simulink model "AS1_Un_Balanced_load_7bus"  (R2021a)
settings: Solver=ode45  StartTime=0.0  StopTime=1  RelTol=1e-3  EnableMultiTasking=on
undefined symbols (not defined in the file): D11, Delta
libraries: spsDCVoltageSourceLib x12, spsDiodeLib x12, spsSeriesRLCBranchLib x12, spsGroundLib x9, spsThreePhaseTransformerTwoWindingsLib x7, spsBreakerLib x7, spsThreePhaseParallelRLCLoadLib x6, simulink_extras x6, spsThreePhaseSeriesRLCBranchLib x6, dspstat3 x3, spsThreePhaseVIMeasurementLib x3, spsCurrentMeasurementLib x2
settings Model: Creator=Gajanan-pc  LastModifiedBy=sony
settings SolverCC: AlgebraicLoopSolver=TrustRegion
settings DataIOCC: LimitDataPoints=on  SaveFormat=Array  ReturnWorkspaceOutputs=off
settings OptimizationCC: LifeSpan=inf
settings DebuggingCC: MaxConsecutiveZCsMsg=none  SolverPrmCheckMsg=warning  ParameterPrecisionLossMsg=none  SFUnexpectedBacktrackingDiag=warning  SFNoUnconditionalDefaultTransitionDiag=warning  SFExecutionAtInitializationDiag=none  SFMachineParentedDataDiag=warning  ArithmeticOperatorsInVariantConditions=warning
settings HardwareCC: ProdBitPerPointer=32  ProdBitPerSizeT=32  ProdBitPerPtrDiffT=32  ProdLargestAtomicFloat=None  ProdIntDivRoundTo=Undefined  ProdEndianess=Unspecified  ProdWordSize=32  ProdHWDeviceType=32-bit Generic
settings ModelReferenceCC: PropagateSignalLabelsOutOfModel=off
settings SFSimCC: SimUseLocalCustomCode=off  CustomCodeUndefinedFunction=UseInterfaceOnly
settings RTWCC: RTWUseLocalCustomCode=off
settings CodeAppCC: StateflowObjectComments=on
settings GRTTargetCC: TargetLangStandard=C89/C90 (ANSI)
settings ConfigComp: CovMetricSettings=dw  CovSaveCumulativeToWorkspaceVar=on  CovSaveSingleToWorkspaceVar=on  CovExternalEMLEnable=off  CovSFcnEnable=off
settings SimscapeCC: SimscapeNormalizeSystem=off

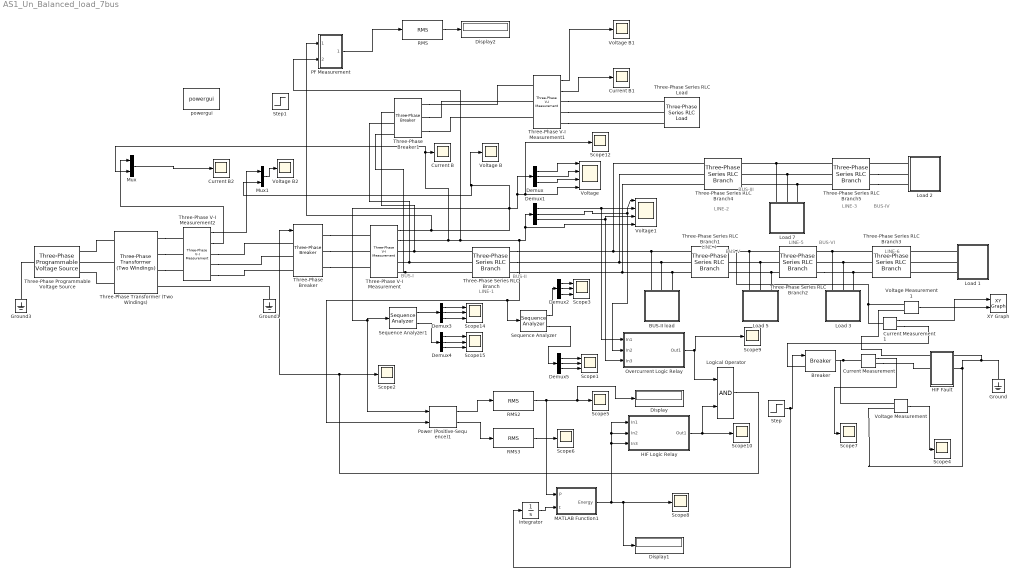
== system AS1_Un_Balanced_load_7bus ==
  note: LINE-1
  note: BUS-I
  note: BUS-II
  note: BUS-III
  note: BUS-IV
  note: BUS-V
  note: BUS-VI
  note: LINE-2
  note: LINE-3
  note: LINE-4
  note: LINE-5
  note: LINE-6
  BUS-II load : Subsystem
  Breaker : spsBreakerLib/Breaker  InitialState=0  SwitchingTimes="[1/50  5/50]"  External=on  BreakerResistance=0.01  SnubberResistance=1e6  SnubberCapacitance=inf  Measurements=Branch voltage and current  MoreParameters=on  NoBreakLoop=off
      settings: SourceProductBaseCode=PS
  Current B : Scope
  Current B1 : Scope
  Current B2 : Scope
  Current Measurement : spsCurrentMeasurementLib/Current Measurement  PhasorSimulation=off  OutputType=Complex  PSBequivalent=0
  Current Measurement1 : spsCurrentMeasurementLib/Current Measurement  PhasorSimulation=off  OutputType=Complex  PSBequivalent=0
  Demux{,1..5} (6 alike) : Demux  Outputs=3
  Display : Display
  Display1 : Display
  Display2 : Display
  Ground : spsGroundLib/Ground  LConnTagsString=a
  Ground1 : spsGroundLib/Ground  LConnTagsString=a
  Ground3 : spsGroundLib/Ground  LConnTagsString=a
  HIF Fault : Subsystem
  HIF Logic Relay : Subsystem  TreatAsAtomicUnit=on
  Integrator : Integrator
  Load 1 : Subsystem
  Load 2 : Subsystem
  Load 3 : Subsystem
  Load 5 : Subsystem
  Load 7 : Subsystem
  Logical Operator : Logic  AllPortsSameDT=off
  MATLAB Function1 : MATLAB Function  TreatAsAtomicUnit=on
  Mux : Mux  Inputs=2
  Mux1 : Mux  Inputs=2
  Overcurrent Logic Relay : Subsystem  TreatAsAtomicUnit=on
  PF Measurement : Subsystem
  Power (Positive-Sequence)1 : spsPowerPositiveSequenceLib/Power (Positive-Sequence)  Freq=50  Vinit=[0, 0]  Iinit=[0, 0]  Ts=0
      link override Sequence Analyzer: Freq=50  seq=Negative
      link override Sequence Analyzer1: Freq=50  seq=Zero
      settings: SourceProductBaseCode=PS
  RMS : dspstat3/RMS  run=off  directionMode=Each column  dimension=1  InputProcessing=Columns as channels (frame based)  reset_popup=None
  RMS2 : dspstat3/RMS  run=off  directionMode=Each column  dimension=1  InputProcessing=Columns as channels (frame based)  reset_popup=None
  RMS3 : dspstat3/RMS  run=off  directionMode=Each column  dimension=1  InputProcessing=Columns as channels (frame based)  reset_popup=None
  Scope{1,3,14..15} (4 alike) : Scope  NumInputPorts=3
  Scope{2,4..10,12} (9 alike) : Scope
  Sequence Analyzer : spsSequenceAnalyzerLib/Sequence Analyzer  Freq=50  n=1  seq=Positive Negative Zero  InInit=[1, 0]  Ts=0
      link override Fourier_A: Freq=50
      link override Fourier_B: Freq=50
      link override Fourier_C: Freq=50
      settings: SourceProductBaseCode=PS
  Sequence Analyzer1 : spsSequenceAnalyzerLib/Sequence Analyzer  Freq=50  n=1  seq=Positive Negative Zero  InInit=[1, 0]  Ts=0
      link override Fourier_A: Freq=50
      link override Fourier_B: Freq=50
      link override Fourier_C: Freq=50
      settings: SourceProductBaseCode=PS
  Step : Step  Time=0.9  SampleTime=0.1  ZeroCross=off
  Step1 : Step  Time=0.8  SampleTime=0.1  ZeroCross=off
  Three-Phase Programmable Voltage Source : spsThreePhaseProgrammableVoltageSourceLib/Three-Phase Programmable Voltage Source  PositiveSequence="[33e3  0 50]"  VariationEntity=None  VariationType=Table of time-amplitude pairs  VariationTypeAlt=Step  VariationStep=0.5  VariationRate=10  VariationMagnitude=0.3  VariationFrequency=2  VariationTiming=[.01 .05 1]  VariationPhaseA=off  Amplitudes=[1 0.8 1.2 1.0]  TimeValues=[0 0.1 0.15 0.2]  HarmonicGeneration=off  HarmonicA=[3 0.2 -25 0]  HarmonicB=[2 0.15 35 2]  Timing="[0.05  3]"  BusType=PQ  Pref=5e6  Qref=0  Qmin=0.5e6  Qmax=0
  Three-Phase Series RLC Branch : spsThreePhaseSeriesRLCBranchLib/Three-Phase Series RLC Branch  LConnTagsString=A|B|C  RConnTagsString=A|B|C  BranchType=RL  Resistance=0.2232  Inductance=0.012  Capacitance=0  Measurements=None
  Three-Phase Series RLC Branch1 : spsThreePhaseSeriesRLCBranchLib/Three-Phase Series RLC Branch  LConnTagsString=A|B|C  RConnTagsString=A|B|C  BranchType=RL  Resistance=0.9207  Inductance=0.0495  Capacitance=0  Measurements=None
  Three-Phase Series RLC Branch2 : spsThreePhaseSeriesRLCBranchLib/Three-Phase Series RLC Branch  LConnTagsString=A|B|C  RConnTagsString=A|B|C  BranchType=RL  Resistance=0.6138  Inductance=0.33  Capacitance=0  Measurements=None
  Three-Phase Series RLC Branch3 : spsThreePhaseSeriesRLCBranchLib/Three-Phase Series RLC Branch  LConnTagsString=A|B|C  RConnTagsString=A|B|C  BranchType=RL  Resistance=1.602  Inductance=0.057  Capacitance=0  Measurements=None
  Three-Phase Series RLC Branch4 : spsThreePhaseSeriesRLCBranchLib/Three-Phase Series RLC Branch  LConnTagsString=A|B|C  RConnTagsString=A|B|C  BranchType=RL  Resistance=0.7812  Inductance=0.042  Capacitance=0  Measurements=None
  Three-Phase Series RLC Branch5 : spsThreePhaseSeriesRLCBranchLib/Three-Phase Series RLC Branch  LConnTagsString=A|B|C  RConnTagsString=A|B|C  BranchType=RL  Resistance=1.1997  Inductance=0.0645  Capacitance=0  Measurements=None
  Three-Phase Series RLC Load : spsThreePhaseSeriesRLCLoadLib/Three-Phase Series RLC Load  LConnTagsString=A|B|C  Configuration=Y (floating)  NominalVoltage=12e3  Vabc=[1e3 1e3 1e3]  Vabcp=[1e3 1e3 1e3]  NominalFrequency=50  UnbalancedPower=off  ActivePower=0  InductivePower=18e3  CapacitivePower=1800e3  Pabc=[10e3 9e3 11e3]  QLabc=[100 90 110]  QCabc=[100 90 110]  Pabcp=[10e3 9e3 11e3]  QLabcp=[100 90 110]  QCabcp=[100 90 110]  Measurements=Branch voltages and currents  LoadType=constant Z
  Three-Phase Transformer (Two Windings) : spsThreePhaseTransformerTwoWindingsLib/Three-Phase Transformer (Two Windings)  Winding1Connection=Delta (D11)  Winding2Connection=Yn  CoreType=Three-limb core (core-type)  SetSaturation=off  Hysteresis=off  DataFile='hysteresis'  SetInitialFlux=off  Measurements=None  UNITS=pu  NominalPower=[ 10e6 , 50 ]  Winding1=[33e3 , 0.002 , 0.08 ]  Winding2=[11e3 , 0.002 , 0.08 ]  Rm=500  Lm=500  L0=0.5  Saturation=[ 0,0 ; 0.0024,1.2 ; 1.0,1.52 ]  InitialFluxes=[-0.84855560977397 0.870082768362299 -0.0215271585931069]  BreakLoop=off  DiscreteSolver=Trapezoidal iterative  DataType=off  TransfoNumber=1
  Three-Phase V-I Measurement : spsThreePhaseVIMeasurementLib/Three-Phase V-I Measurement  VoltageMeasurement=phase-to-phase  SetLabelV=off  LabelV=Vabc  Vpu=off  VpuLL=off  CurrentMeasurement=yes  SetLabelI=off  LabelI=Iabc  Ipu=off  Pbase=100e6  Vbase=11e3  OutputType=Complex  PhasorSimulation=off  PSBequivalent=0
  Three-Phase V-I Measurement1 : spsThreePhaseVIMeasurementLib/Three-Phase V-I Measurement  VoltageMeasurement=phase-to-phase  SetLabelV=off  LabelV=Vabc  Vpu=off  VpuLL=off  CurrentMeasurement=yes  SetLabelI=off  LabelI=Iabc  Ipu=off  Pbase=100e6  Vbase=11e3  OutputType=Complex  PhasorSimulation=off  PSBequivalent=0
  Three-Phase V-I Measurement2 : spsThreePhaseVIMeasurementLib/Three-Phase V-I Measurement  VoltageMeasurement=phase-to-phase  SetLabelV=off  LabelV=Vabc  Vpu=off  VpuLL=off  CurrentMeasurement=yes  SetLabelI=off  LabelI=Iabc  Ipu=off  Pbase=100e6  Vbase=11e3  OutputType=Complex  PhasorSimulation=off  PSBequivalent=0
  Three-Phase Breaker : spsThreePhaseBreakerLib/Three-Phase Breaker  InitialState=closed  SwitchA=on  SwitchB=on  SwitchC=on  SwitchTimes=[1/50 5/50]  External=on  BreakerResistance=0.01  SnubberResistance=1e6  SnubberCapacitance=inf  Measurements=Breaker voltages and currents
  Three-Phase Breaker1 : spsThreePhaseBreakerLib/Three-Phase Breaker  InitialState=closed  SwitchA=on  SwitchB=on  SwitchC=on  SwitchTimes=[1/50 5/50]  External=on  BreakerResistance=0.01  SnubberResistance=1e6  SnubberCapacitance=inf  Measurements=Breaker voltages and currents
  Voltage : Scope  NumInputPorts=4
  Voltage B : Scope
  Voltage B1 : Scope
  Voltage B2 : Scope
  Voltage Measurement : spsVoltageMeasurementLib/Voltage Measurement  PhasorSimulation=off  OutputType=Complex  PSBequivalent=0
  Voltage Measurement1 : spsVoltageMeasurementLib/Voltage Measurement  PhasorSimulation=off  OutputType=Complex  PSBequivalent=0
  Voltage1 : Scope  NumInputPorts=4
  XY Graph : simulink/Sinks/XY Graph  xmin=-100  xmax=100  ymin=-7000  ymax=7000  st=-1
  powergui : spspowerguiLib/powergui  Priority=1  SimulationMode=Discrete  SampleTime=50e-6  frequency=60  Iterations=50  frequencyindice=0  Pbase=100e6  ErrMax=0.0001  UnitsV=kV  UnitsW=MW  buscounter=0  FunctionMessages=off  echomessages=off  EnableUseOfTLC=off  CurrentSourceSwitches=off  DisableSnubberDevices=off  DisableRonSwitches=off  DisableVfSwitches=off  DisplayEquations=off  AutomaticDiscreteSolvers=off  SolverType=Backward Euler  Interpol=off  ExternalGateDelay=off  methode=off  Ts=0  x0status=blocks  SPID=off  SwTol=0  HookPort=off  NonlinearTolerance=0  nMaxIteration=15  ContinueOnMaxIteration=off  RestoreLinks=warning  ResistiveCurrentMeasurement=off  Frange=[0:2:500]  Ylog=off  Xlog=on  ShowGrid=off  save=off  variable=ZData  structure=0  ZoomFFT=off  StartTime=0.0  cycles=1  DisplayStyle=1  fundamental=60  FreqAxis=off  MaxFrequency=1000  frequencyindicesteady=1  RmsSteady=1  display=off
  wires:
  Demux1/3 -> Voltage1/3, Overcurrent Logic Relay/3(In3)
  Demux/1 -> Voltage/1
  Demux/2 -> Voltage/2
  Demux/3 -> Voltage/3
  Demux1/2 -> Voltage1/2, Overcurrent Logic Relay/2(In2)
  Three-Phase V-I Measurement/1 -> PF Measurement/1(In1), Mux1/2, Voltage B/1, Power (Positive-Sequence)1/1, Sequence Analyzer1/1, Scope12/1, Voltage/4, Demux/1
  Overcurrent Logic Relay/1(Out1) -> Logical Operator/1, Scope9/1
  Step/1 -> Integrator/1, Breaker/1
  Voltage Measurement/1 -> Scope4/1
  Sequence Analyzer/1 -> Demux2/1
  HIF Logic Relay/1(Out1) -> Logical Operator/2, Scope10/1
  Demux1/1 -> Voltage1/1, Overcurrent Logic Relay/1(In1)
  Current Measurement/1 -> Scope7/1
  Current Measurement1/1 -> XY Graph/1
  Voltage Measurement1/1 -> XY Graph/2
  Demux2/1 -> Scope3/1
  Sequence Analyzer1/1 -> Demux3/1
  Demux3/1 -> Scope14/1
  Demux3/2 -> Scope14/2
  Demux3/3 -> Scope14/3
  Sequence Analyzer1/2 -> Demux4/1
  Demux4/1 -> Scope15/1
  Demux4/2 -> Scope15/2
  Demux4/3 -> Scope15/3
  Demux2/2 -> Scope3/2
  Demux5/1 -> Scope1/1
  Demux5/2 -> Scope1/2
  Demux5/3 -> Scope1/3
  Sequence Analyzer/2 -> Demux5/1
  Demux2/3 -> Scope3/3
  Power (Positive-Sequence)1/1 -> RMS2/1
  RMS2/1 -> MATLAB Function1/1(P), Display/1, Scope5/1
  Power (Positive-Sequence)1/2 -> RMS3/1
  RMS3/1 -> Scope6/1
  Integrator/1 -> MATLAB Function1/2(t)
  MATLAB Function1/1(Energy) -> HIF Logic Relay/3(In3), HIF Logic Relay/2(In2), HIF Logic Relay/1(In1), Scope8/1, Display1/1
  Three-Phase V-I Measurement/2 -> Mux/2, Current B/1, PF Measurement/2(In2), Sequence Analyzer/1, Power (Positive-Sequence)1/2, Demux1/1, Voltage1/4
  Logical Operator/1 -> Three-Phase Breaker/1, Scope2/1
  Three-Phase V-I Measurement1/1 -> Voltage B1/1
  Three-Phase V-I Measurement1/2 -> Current B1/1
  RMS/1 -> Display2/1
  PF Measurement/1(Out1) -> RMS/1
  Mux/1 -> Current B2/1
  Three-Phase V-I Measurement2/2 -> Mux/1
  Three-Phase V-I Measurement2/1 -> Mux1/1
  Mux1/1 -> Voltage B2/1
  connections:
  Three-Phase Series RLC Branch3/LConn2 -- Load 3/LConn2 -- Three-Phase Series RLC Branch2/RConn2
  Three-Phase Series RLC Branch2/RConn3 -- Load 3/LConn3 -- Three-Phase Series RLC Branch3/LConn3
  Voltage Measurement/LConn1 -- Breaker/RConn1 -- Current Measurement/LConn1
  Voltage Measurement/LConn2 -- HIF Fault/RConn1 -- Voltage Measurement1/LConn2 -- Ground/LConn1
  Three-Phase Series RLC Branch/LConn2 -- Three-Phase Breaker1/LConn2 -- Three-Phase V-I Measurement/RConn2
  Three-Phase Breaker/RConn2 -- Three-Phase V-I Measurement/LConn2
  Current Measurement1/RConn1 -- Breaker/LConn1
  Three-Phase Series RLC Branch/RConn3 -- BUS-II load/LConn3 -- Three-Phase Series RLC Branch1/LConn3 -- Three-Phase Series RLC Branch4/LConn3
  Three-Phase Series RLC Branch/LConn3 -- Three-Phase Breaker1/LConn3 -- Three-Phase V-I Measurement/RConn3
  Three-Phase Breaker/RConn1 -- Three-Phase V-I Measurement/LConn1
  Three-Phase Breaker/RConn3 -- Three-Phase V-I Measurement/LConn3
  Current Measurement/RConn1 -- HIF Fault/LConn1
  Three-Phase Series RLC Branch5/LConn2 -- Load 7/LConn2 -- Three-Phase Series RLC Branch4/RConn2
  Three-Phase Series RLC Branch5/LConn3 -- Load 7/LConn3 -- Three-Phase Series RLC Branch4/RConn3
  Three-Phase Series RLC Branch/LConn1 -- Three-Phase Breaker1/LConn1 -- Three-Phase V-I Measurement/RConn1
  Three-Phase Series RLC Branch1/RConn3 -- Load 5/LConn3 -- Three-Phase Series RLC Branch2/LConn3
  Three-Phase Series RLC Branch/RConn1 -- BUS-II load/LConn1 -- Three-Phase Series RLC Branch1/LConn1 -- Three-Phase Series RLC Branch4/LConn1
  Three-Phase V-I Measurement1/RConn1 -- Three-Phase Series RLC Load/LConn1
  Three-Phase V-I Measurement1/RConn2 -- Three-Phase Series RLC Load/LConn2
  Three-Phase V-I Measurement1/RConn3 -- Three-Phase Series RLC Load/LConn3
  Three-Phase Breaker1/RConn1 -- Three-Phase V-I Measurement1/LConn1
  Three-Phase Breaker1/RConn2 -- Three-Phase V-I Measurement1/LConn2
  Three-Phase Breaker1/RConn3 -- Three-Phase V-I Measurement1/LConn3
  Three-Phase Series RLC Branch2/LConn2 -- Load 5/LConn2 -- Three-Phase Series RLC Branch1/RConn2
  Three-Phase Series RLC Branch1/LConn2 -- BUS-II load/LConn2 -- Three-Phase Series RLC Branch4/LConn2 -- Three-Phase Series RLC Branch/RConn2
  Three-Phase Transformer (Two Windings)/LConn1 -- Three-Phase Programmable Voltage Source/RConn1
  Three-Phase Transformer (Two Windings)/LConn2 -- Three-Phase Programmable Voltage Source/RConn2
  Three-Phase Transformer (Two Windings)/LConn3 -- Three-Phase Programmable Voltage Source/RConn3
  Three-Phase Programmable Voltage Source/LConn1 -- Ground3/LConn1
  Three-Phase Series RLC Branch5/LConn1 -- Load 7/LConn1 -- Three-Phase Series RLC Branch4/RConn1
  Load 1/LConn2 -- Three-Phase Series RLC Branch3/RConn2
  Load 1/LConn3 -- Three-Phase Series RLC Branch3/RConn3
  Load 1/LConn1 -- Three-Phase Series RLC Branch3/RConn1
  Load 2/LConn1 -- Three-Phase Series RLC Branch5/RConn1
  Three-Phase Series RLC Branch5/RConn2 -- Load 2/LConn2
  Three-Phase Series RLC Branch5/RConn3 -- Load 2/LConn3
  Three-Phase Series RLC Branch3/LConn1 -- Load 3/LConn1 -- Three-Phase Series RLC Branch2/RConn1
  Ground1/LConn1 -- Three-Phase Transformer (Two Windings)/RConn4
  Load 5/LConn1 -- Voltage Measurement1/LConn1 -- Current Measurement1/LConn1 -- Three-Phase Series RLC Branch1/RConn1 -- Three-Phase Series RLC Branch2/LConn1
  Three-Phase Transformer (Two Windings)/RConn1 -- Three-Phase V-I Measurement2/LConn1
  Three-Phase Transformer (Two Windings)/RConn2 -- Three-Phase V-I Measurement2/LConn2
  Three-Phase Transformer (Two Windings)/RConn3 -- Three-Phase V-I Measurement2/LConn3
  Three-Phase V-I Measurement2/RConn1 -- Three-Phase Breaker/LConn1
  Three-Phase V-I Measurement2/RConn2 -- Three-Phase Breaker/LConn2
  Three-Phase V-I Measurement2/RConn3 -- Three-Phase Breaker/LConn3

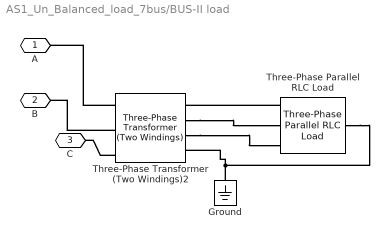
== system AS1_Un_Balanced_load_7bus/BUS-II load ==
  Ground : spsGroundLib/Ground  LConnTagsString=a
  Three-Phase Parallel RLC Load : spsThreePhaseParallelRLCLoadLib/Three-Phase Parallel RLC Load  LConnTagsString=A|B|C  RConnTagsString=N  Configuration=Y (neutral)  NominalVoltage=[248 248 248]  Vabc=[248 248 248]  Vabcp=[1e3 1e3 1e3]  NominalFrequency=50  UnbalancedPower=on  ActivePower=10e3  InductivePower=100  CapacitivePower=100  Pabc=[120e3 144e3 40e3]  QLabc=[23.33e3 16.66e3 10e3]  QCabc=[0 0 0]  Pabcp=[10e3 9e3 11e3]  QLabcp=[100 90 110]  QCabcp=[100 90 110]  Measurements=Branch voltages and currents  LoadType=constant Z
  Three-Phase Transformer (Two Windings)2 : spsThreePhaseTransformerTwoWindingsLib/Three-Phase Transformer (Two Windings)  Winding1Connection=Delta (D11)  Winding2Connection=Yn  CoreType=Three-limb core (core-type)  SetSaturation=off  Hysteresis=off  DataFile='hysteresis'  SetInitialFlux=off  Measurements=All measurements (V I Fluxes)  UNITS=pu  NominalPower=[ 0.5e6 , 50 ]  Winding1=[11e3 , 0.002 , 0.08 ]  Winding2=[433 , 0.002 , 0.08 ]  Rm=250  Lm=250  L0=0.5  Saturation=[ 0,0 ; 0.0024,1.2 ; 1.0,1.52 ]  InitialFluxes=[-0.256778366744012 0.860170931387357 -0.584038315133465]  BreakLoop=off  DiscreteSolver=Trapezoidal iterative  DataType=off  TransfoNumber=1
  A : PMIOPort  Side=Left
  B : PMIOPort  Port=2  Side=Left
  C : PMIOPort  Port=3  Side=Left
  connections:
  Three-Phase Transformer (Two Windings)2/LConn1 -- A/RConn1
  Three-Phase Transformer (Two Windings)2/LConn3 -- C/RConn1
  Three-Phase Transformer (Two Windings)2/LConn2 -- B/RConn1
  Ground/LConn1 -- Three-Phase Parallel RLC Load/RConn1 -- Three-Phase Transformer (Two Windings)2/RConn4
  Three-Phase Parallel RLC Load/LConn1 -- Three-Phase Transformer (Two Windings)2/RConn1
  Three-Phase Transformer (Two Windings)2/RConn2 -- Three-Phase Parallel RLC Load/LConn2
  Three-Phase Transformer (Two Windings)2/RConn3 -- Three-Phase Parallel RLC Load/LConn3

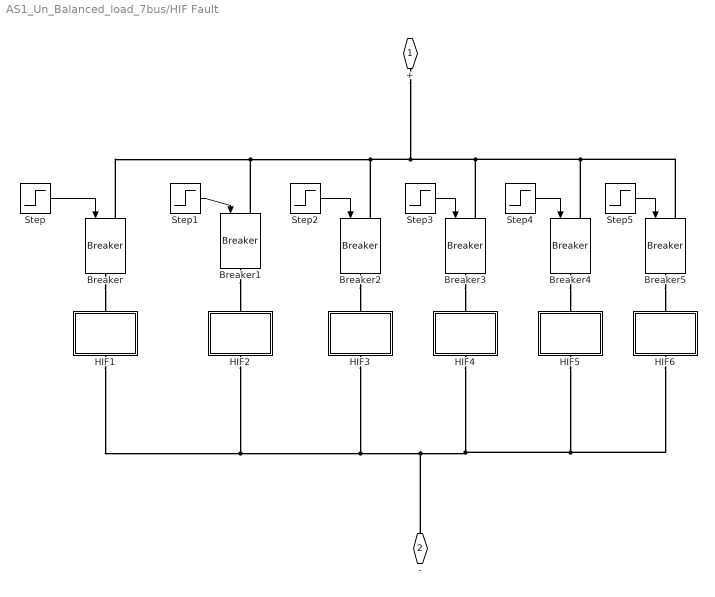
== system AS1_Un_Balanced_load_7bus/HIF Fault ==
  Breaker{,1..5} (6 alike) : spsBreakerLib/Breaker  InitialState=0  SwitchingTimes="[1/50  5/50]"  External=on  BreakerResistance=0.01  SnubberResistance=1e6  SnubberCapacitance=inf  Measurements=Branch voltage and current  MoreParameters=on  NoBreakLoop=off
      settings: SourceProductBaseCode=PS
  HIF1 : Subsystem
  HIF2 : Subsystem
  HIF3 : Subsystem
  HIF4 : Subsystem
  HIF5 : Subsystem
  HIF6 : Subsystem
  Step : Step  Time=0.01  SampleTime=0.001  ZeroCross=off
  Step1 : Step  Time=0.12  SampleTime=0.001  ZeroCross=off
  Step2 : Step  Time=0.14  SampleTime=0.001  ZeroCross=off
  Step3 : Step  Time=0.16  SampleTime=0.001  ZeroCross=off
  Step4 : Step  Time=0.18  SampleTime=0.001  VectorParams1D=off
  Step5 : Step  Time=0.2  SampleTime=0.001  VectorParams1D=off
  + : PMIOPort  Side=Left
  - : PMIOPort  Port=2  Side=Right
  wires:
  Step4/1 -> Breaker4/1
  Step1/1 -> Breaker1/1
  Step2/1 -> Breaker2/1
  Step3/1 -> Breaker3/1
  Step/1 -> Breaker/1
  Step5/1 -> Breaker5/1
  connections:
  Breaker/LConn1 -- Breaker1/LConn1 -- Breaker2/LConn1 -- Breaker5/LConn1 -- Breaker4/LConn1 -- Breaker3/LConn1 -- +/RConn1
  Breaker/RConn1 -- HIF1/LConn1
  Breaker4/RConn1 -- HIF5/LConn1
  Breaker5/RConn1 -- HIF6/LConn1
  Breaker3/RConn1 -- HIF4/LConn1
  Breaker2/RConn1 -- HIF3/LConn1
  HIF5/RConn1 -- HIF6/RConn1 -- HIF4/RConn1 -- HIF3/RConn1 -- HIF2/RConn1 -- HIF1/RConn1 -- -/RConn1
  Breaker1/RConn1 -- HIF2/LConn1

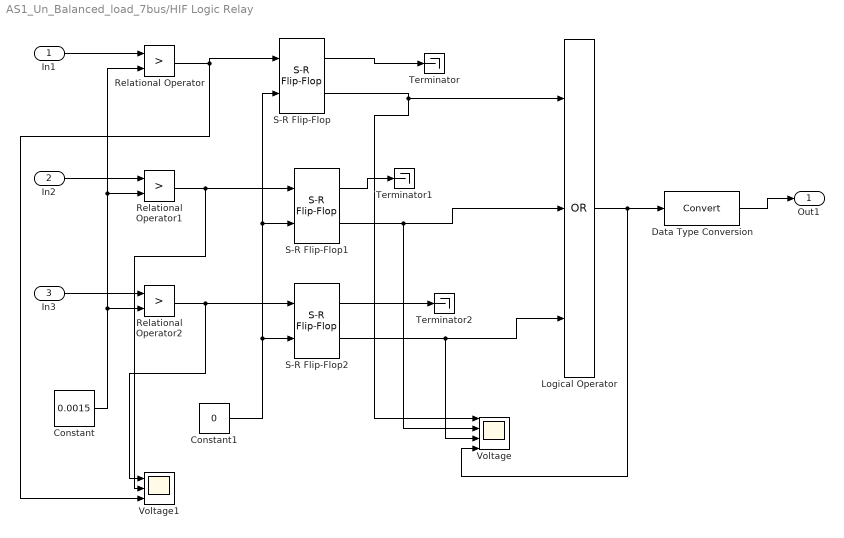
== system AS1_Un_Balanced_load_7bus/HIF Logic Relay ==
  In1 : Inport
  In2 : Inport  Port=2
  In3 : Inport  Port=3
  Constant : Constant  Value=0.0015  VectorParams1D=off  OutDataTypeStr=Inherit: Inherit via back propagation  LockScale=on
  Constant1 : Constant  Value=0  VectorParams1D=off  OutDataTypeStr=Inherit: Inherit via back propagation  LockScale=on
  Data Type Conversion : DataTypeConversion
  Logical Operator : Logic  Operator=OR  Inputs=3  AllPortsSameDT=off
  Relational Operator : RelationalOperator  Operator=>  RndMeth=Nearest
  Relational Operator1 : RelationalOperator  Operator=>  RndMeth=Nearest
  Relational Operator2 : RelationalOperator  Operator=>  RndMeth=Nearest
  S-R Flip-Flop : simulink_extras/Flip Flops/S-R Flip-Flop  initial_condition=0
  S-R Flip-Flop1 : simulink_extras/Flip Flops/S-R Flip-Flop  initial_condition=0
  S-R Flip-Flop2 : simulink_extras/Flip Flops/S-R Flip-Flop  initial_condition=0
  Terminator : Terminator
  Terminator1 : Terminator
  Terminator2 : Terminator
  Voltage : Scope  NumInputPorts=4
  Voltage1 : Scope  NumInputPorts=3
  Out1 : Outport  VectorParamsAs1DForOutWhenUnconnected=off
  wires:
  In1/1 -> Relational Operator/1
  In2/1 -> Relational Operator1/1
  In3/1 -> Relational Operator2/1
  Constant/1 -> Relational Operator2/2, Relational Operator1/2, Relational Operator/2
  Relational Operator/1 -> Voltage1/3, S-R Flip-Flop/1
  Relational Operator1/1 -> Voltage1/2, S-R Flip-Flop1/1
  Relational Operator2/1 -> Voltage1/1, S-R Flip-Flop2/1
  Constant1/1 -> S-R Flip-Flop2/2, S-R Flip-Flop1/2, S-R Flip-Flop/2
  S-R Flip-Flop/1 -> Terminator/1
  S-R Flip-Flop1/1 -> Terminator1/1
  S-R Flip-Flop2/1 -> Terminator2/1
  S-R Flip-Flop/2 -> Voltage/1, Logical Operator/1
  S-R Flip-Flop1/2 -> Voltage/2, Logical Operator/2
  S-R Flip-Flop2/2 -> Voltage/3, Logical Operator/3
  Data Type Conversion/1 -> Out1/1
  Logical Operator/1 -> Voltage/4, Data Type Conversion/1

== system AS1_Un_Balanced_load_7bus/Load 1 ==
  Ground : spsGroundLib/Ground  LConnTagsString=a
  Three-Phase Parallel RLC Load1 : spsThreePhaseParallelRLCLoadLib/Three-Phase Parallel RLC Load  LConnTagsString=A|B|C  RConnTagsString=N  Configuration=Y (neutral)  NominalVoltage=[248 248 248]  Vabc=[248 248 248]  Vabcp=[1e3 1e3 1e3]  NominalFrequency=50  UnbalancedPower=on  ActivePower=10e3  InductivePower=100  CapacitivePower=100  Pabc=[ 1e3 210.66e3 215.e3 ]  QLabc=[1e3 104e3 66e3]  QCabc=[0 0 0]  Pabcp=[10e3 9e3 11e3]  QLabcp=[100 90 110]  QCabcp=[100 90 110]  Measurements=Branch voltages and currents  LoadType=constant Z
  Three-Phase Transformer (Two Windings)2 : spsThreePhaseTransformerTwoWindingsLib/Three-Phase Transformer (Two Windings)  Winding1Connection=Delta (D11)  Winding2Connection=Yn  CoreType=Three-limb core (core-type)  SetSaturation=off  Hysteresis=off  DataFile='hysteresis'  SetInitialFlux=off  Measurements=All measurements (V I Fluxes)  UNITS=pu  NominalPower=[ 0.5e6 , 50 ]  Winding1=[11e3 , 0.002 , 0.08 ]  Winding2=[433 , 0.002 , 0.08 ]  Rm=250  Lm=250  L0=0.5  Saturation=[ 0,0 ; 0.0024,1.2 ; 1.0,1.52 ]  InitialFluxes=[0.167363107089062 0.0610185437238888 -0.245329692895651]  BreakLoop=off  DiscreteSolver=Trapezoidal iterative  DataType=off  TransfoNumber=1
  A : PMIOPort  Side=Left
  B : PMIOPort  Port=2  Side=Left
  C : PMIOPort  Port=3  Side=Left
  connections:
  Three-Phase Transformer (Two Windings)2/LConn2 -- B/RConn1
  Three-Phase Transformer (Two Windings)2/LConn3 -- C/RConn1
  Three-Phase Transformer (Two Windings)2/LConn1 -- A/RConn1
  Three-Phase Transformer (Two Windings)2/RConn2 -- Three-Phase Parallel RLC Load1/LConn2
  Three-Phase Transformer (Two Windings)2/RConn1 -- Three-Phase Parallel RLC Load1/LConn1
  Three-Phase Transformer (Two Windings)2/RConn3 -- Three-Phase Parallel RLC Load1/LConn3
  Three-Phase Transformer (Two Windings)2/RConn4 -- Three-Phase Parallel RLC Load1/RConn1 -- Ground/LConn1

== system AS1_Un_Balanced_load_7bus/Load 2 ==
  Ground : spsGroundLib/Ground  LConnTagsString=a
  Three-Phase Parallel RLC Load1 : spsThreePhaseParallelRLCLoadLib/Three-Phase Parallel RLC Load  LConnTagsString=A|B|C  RConnTagsString=N  Configuration=Y (neutral)  NominalVoltage=[248 248 248]  Vabc=[248 248 248]  Vabcp=[1e3 1e3 1e3]  NominalFrequency=50  UnbalancedPower=on  ActivePower=10e3  InductivePower=100  CapacitivePower=100  Pabc=[48.33e3 1e3 1e3]  QLabc=[9.33e3 1e3 1e3]  QCabc=[0 0 0]  Pabcp=[10e3 9e3 11e3]  QLabcp=[100 90 110]  QCabcp=[100 90 110]  Measurements=Branch voltages and currents  LoadType=constant Z
  Three-Phase Transformer (Two Windings)2 : spsThreePhaseTransformerTwoWindingsLib/Three-Phase Transformer (Two Windings)  Winding1Connection=Delta (D11)  Winding2Connection=Yn  CoreType=Three-limb core (core-type)  SetSaturation=off  Hysteresis=off  DataFile='hysteresis'  SetInitialFlux=off  Measurements=All measurements (V I Fluxes)  UNITS=pu  NominalPower=[0.5e3 , 50 ]  Winding1=[11e3 , 0.002 , 0.08 ]  Winding2=[433 , 0.002 , 0.08 ]  Rm=250  Lm=250  L0=0.5  Saturation=[ 0,0 ; 0.0024,1.2 ; 1.0,1.52 ]  InitialFluxes=[-0.093644263507764 0.838815084304348 -0.653451497613207]  BreakLoop=off  DiscreteSolver=Trapezoidal iterative  DataType=off  TransfoNumber=1
  A : PMIOPort  Side=Left
  B : PMIOPort  Port=2  Side=Left
  C : PMIOPort  Port=3  Side=Left
  connections:
  Three-Phase Transformer (Two Windings)2/LConn2 -- B/RConn1
  Three-Phase Transformer (Two Windings)2/LConn3 -- C/RConn1
  Three-Phase Transformer (Two Windings)2/LConn1 -- A/RConn1
  Three-Phase Transformer (Two Windings)2/RConn3 -- Three-Phase Parallel RLC Load1/LConn3
  Three-Phase Parallel RLC Load1/LConn1 -- Three-Phase Transformer (Two Windings)2/RConn1
  Three-Phase Transformer (Two Windings)2/RConn2 -- Three-Phase Parallel RLC Load1/LConn2
  Ground/LConn1 -- Three-Phase Parallel RLC Load1/RConn1 -- Three-Phase Transformer (Two Windings)2/RConn4

== system AS1_Un_Balanced_load_7bus/Load 3 ==
  Ground : spsGroundLib/Ground  LConnTagsString=a
  Three-Phase Parallel RLC Load2 : spsThreePhaseParallelRLCLoadLib/Three-Phase Parallel RLC Load  LConnTagsString=A|B|C  RConnTagsString=N  Configuration=Y (neutral)  NominalVoltage=[248 248 248]  Vabc=[248 248 248]  Vabcp=[1e3 1e3 1e3]  NominalFrequency=50  UnbalancedPower=on  ActivePower=10e3  InductivePower=100  CapacitivePower=100  Pabc=[144e3 125.66e3 141.66e3]  QLabc=[27.33e3 31e3 34.33e3]  QCabc=[0 0 0]  Pabcp=[10e3 9e3 11e3]  QLabcp=[100 90 110]  QCabcp=[100 90 110]  Measurements=Branch voltages and currents  LoadType=constant Z
  Three-Phase Transformer (Two Windings)2 : spsThreePhaseTransformerTwoWindingsLib/Three-Phase Transformer (Two Windings)  Winding1Connection=Delta (D11)  Winding2Connection=Yn  CoreType=Three-limb core (core-type)  SetSaturation=off  Hysteresis=off  DataFile='hysteresis'  SetInitialFlux=off  Measurements=All measurements (V I Fluxes)  UNITS=pu  NominalPower=[ 0.5e6 , 50 ]  Winding1=[11e3 , 0.002 , 0.08 ]  Winding2=[ 433 , 0.002 , 0.08 ]  Rm=250  Lm=250  L0=0.5  Saturation=[ 0,0 ; 0.0024,1.2 ; 1.0,1.52 ]  InitialFluxes=[0.177589955789988 0.125733120517853 -0.299711964168377]  BreakLoop=off  DiscreteSolver=Trapezoidal iterative  DataType=off  TransfoNumber=1
  A : PMIOPort  Side=Left
  B : PMIOPort  Port=2  Side=Left
  C : PMIOPort  Port=3  Side=Left
  connections:
  Three-Phase Transformer (Two Windings)2/LConn2 -- B/RConn1
  Three-Phase Transformer (Two Windings)2/LConn3 -- C/RConn1
  Three-Phase Transformer (Two Windings)2/LConn1 -- A/RConn1
  Three-Phase Parallel RLC Load2/RConn1 -- Ground/LConn1 -- Three-Phase Transformer (Two Windings)2/RConn4
  Three-Phase Parallel RLC Load2/LConn1 -- Three-Phase Transformer (Two Windings)2/RConn1
  Three-Phase Transformer (Two Windings)2/RConn2 -- Three-Phase Parallel RLC Load2/LConn2
  Three-Phase Transformer (Two Windings)2/RConn3 -- Three-Phase Parallel RLC Load2/LConn3

== system AS1_Un_Balanced_load_7bus/Load 5 ==
  Ground : spsGroundLib/Ground  LConnTagsString=a
  Three-Phase Parallel RLC Load1 : spsThreePhaseParallelRLCLoadLib/Three-Phase Parallel RLC Load  LConnTagsString=A|B|C  RConnTagsString=N  Configuration=Y (neutral)  NominalVoltage=[248 248 248]  Vabc=[248 248 248]  Vabcp=[1e3 1e3 1e3]  NominalFrequency=50  UnbalancedPower=on  ActivePower=10e3  InductivePower=100  CapacitivePower=100  Pabc=[244e3 115e3 75e3]  QLabc=[37.33e3 32.66e3 17.66e3]  QCabc=[0 0 0]  Pabcp=[10e3 9e3 11e3]  QLabcp=[100 90 110]  QCabcp=[100 90 110]  Measurements=Branch voltages and currents  LoadType=constant Z
  Three-Phase Transformer (Two Windings)2 : spsThreePhaseTransformerTwoWindingsLib/Three-Phase Transformer (Two Windings)  Winding1Connection=Delta (D11)  Winding2Connection=Yn  CoreType=Three-limb core (core-type)  SetSaturation=off  Hysteresis=off  DataFile='hysteresis'  SetInitialFlux=off  Measurements=All measurements (V I Fluxes)  UNITS=pu  NominalPower=[ 0.5e6 , 50 ]  Winding1=[ 11e3 , 0.002 , 0.08 ]  Winding2=[ 433 , 0.002 , 0.08 ]  Rm=250  Lm=250  L0=0.5  Saturation=[ 0,0 ; 0.0024,1.2 ; 1.0,1.52 ]  InitialFluxes=[-0.0247540799705537 0.677855009969254 -0.599270009227358]  BreakLoop=off  DiscreteSolver=Trapezoidal iterative  DataType=off  TransfoNumber=1
  A : PMIOPort  Side=Left
  B : PMIOPort  Port=2  Side=Left
  C : PMIOPort  Port=3  Side=Left
  connections:
  Three-Phase Transformer (Two Windings)2/LConn1 -- A/RConn1
  Three-Phase Transformer (Two Windings)2/LConn3 -- C/RConn1
  Three-Phase Transformer (Two Windings)2/LConn2 -- B/RConn1
  Three-Phase Parallel RLC Load1/LConn1 -- Three-Phase Transformer (Two Windings)2/RConn1
  Three-Phase Transformer (Two Windings)2/RConn2 -- Three-Phase Parallel RLC Load1/LConn2
  Three-Phase Transformer (Two Windings)2/RConn3 -- Three-Phase Parallel RLC Load1/LConn3
  Three-Phase Parallel RLC Load1/RConn1 -- Three-Phase Transformer (Two Windings)2/RConn4 -- Ground/LConn1

== system AS1_Un_Balanced_load_7bus/Load 7 ==
  Ground : spsGroundLib/Ground  LConnTagsString=a
  Three-Phase Parallel RLC Load1 : spsThreePhaseParallelRLCLoadLib/Three-Phase Parallel RLC Load  LConnTagsString=A|B|C  RConnTagsString=N  Configuration=Y (neutral)  NominalVoltage=[248 248 248]  Vabc=[248 248 248]  Vabcp=[1e3 1e3 1e3]  NominalFrequency=50  UnbalancedPower=on  ActivePower=10e3  InductivePower=100  CapacitivePower=100  Pabc=[48.33e3 214.33e3 148.33e3]  QLabc=[3.33e3 33.33e3 22.33e3]  QCabc=[0 0 0]  Pabcp=[10e3 9e3 11e3]  QLabcp=[100 90 110]  QCabcp=[100 90 110]  Measurements=Branch voltages and currents  LoadType=constant Z
  Three-Phase Transformer (Two Windings)2 : spsThreePhaseTransformerTwoWindingsLib/Three-Phase Transformer (Two Windings)  Winding1Connection=Delta (D11)  Winding2Connection=Yn  CoreType=Three-limb core (core-type)  SetSaturation=off  Hysteresis=off  DataFile='hysteresis'  SetInitialFlux=off  Measurements=All measurements (V I Fluxes)  UNITS=SI  NominalPower=[0.5e6 , 50 ]  Winding1=[11e3 0.002 0.08]  Winding2=[433 0.002 0.08]  Rm=250  Lm=250  L0=0.36108  Saturation=[0 0;0.16456 59.421;68.568 75.266]  InitialFluxes=[-5.25282919688326 40.1491552037539 -34.8961082612815]  BreakLoop=off  DiscreteSolver=Trapezoidal iterative  DataType=on  TransfoNumber=1
  A : PMIOPort  Side=Left
  B : PMIOPort  Port=2  Side=Left
  C : PMIOPort  Port=3  Side=Left
  connections:
  Three-Phase Transformer (Two Windings)2/LConn2 -- B/RConn1
  Three-Phase Transformer (Two Windings)2/LConn3 -- C/RConn1
  Three-Phase Transformer (Two Windings)2/LConn1 -- A/RConn1
  Three-Phase Parallel RLC Load1/LConn1 -- Three-Phase Transformer (Two Windings)2/RConn1
  Three-Phase Transformer (Two Windings)2/RConn2 -- Three-Phase Parallel RLC Load1/LConn2
  Three-Phase Transformer (Two Windings)2/RConn3 -- Three-Phase Parallel RLC Load1/LConn3
  Three-Phase Parallel RLC Load1/RConn1 -- Ground/LConn1 -- Three-Phase Transformer (Two Windings)2/RConn4

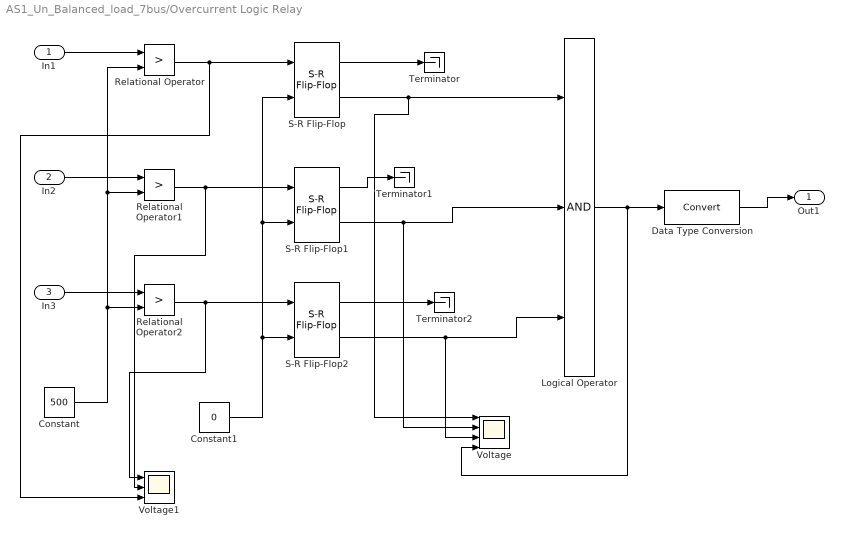
== system AS1_Un_Balanced_load_7bus/Overcurrent Logic Relay ==
  In1 : Inport
  In2 : Inport  Port=2
  In3 : Inport  Port=3
  Constant : Constant  Value=500  VectorParams1D=off  OutDataTypeStr=Inherit: Inherit via back propagation  LockScale=on
  Constant1 : Constant  Value=0  VectorParams1D=off  OutDataTypeStr=Inherit: Inherit via back propagation  LockScale=on
  Data Type Conversion : DataTypeConversion
  Logical Operator : Logic  Inputs=3  AllPortsSameDT=off
  Relational Operator : RelationalOperator  Operator=>  RndMeth=Nearest
  Relational Operator1 : RelationalOperator  Operator=>  RndMeth=Nearest
  Relational Operator2 : RelationalOperator  Operator=>  RndMeth=Nearest
  S-R Flip-Flop : simulink_extras/Flip Flops/S-R Flip-Flop  initial_condition=0
  S-R Flip-Flop1 : simulink_extras/Flip Flops/S-R Flip-Flop  initial_condition=0
  S-R Flip-Flop2 : simulink_extras/Flip Flops/S-R Flip-Flop  initial_condition=0
  Terminator : Terminator
  Terminator1 : Terminator
  Terminator2 : Terminator
  Voltage : Scope  NumInputPorts=4
  Voltage1 : Scope  NumInputPorts=3
  Out1 : Outport  VectorParamsAs1DForOutWhenUnconnected=off
  wires:
  In1/1 -> Relational Operator/1
  In2/1 -> Relational Operator1/1
  In3/1 -> Relational Operator2/1
  Constant/1 -> Relational Operator2/2, Relational Operator1/2, Relational Operator/2
  Relational Operator/1 -> Voltage1/3, S-R Flip-Flop/1
  Relational Operator1/1 -> Voltage1/2, S-R Flip-Flop1/1
  Relational Operator2/1 -> Voltage1/1, S-R Flip-Flop2/1
  Constant1/1 -> S-R Flip-Flop2/2, S-R Flip-Flop1/2, S-R Flip-Flop/2
  S-R Flip-Flop/1 -> Terminator/1
  S-R Flip-Flop1/1 -> Terminator1/1
  S-R Flip-Flop2/1 -> Terminator2/1
  S-R Flip-Flop/2 -> Voltage/1, Logical Operator/1
  S-R Flip-Flop1/2 -> Voltage/2, Logical Operator/2
  S-R Flip-Flop2/2 -> Voltage/3, Logical Operator/3
  Data Type Conversion/1 -> Out1/1
  Logical Operator/1 -> Voltage/4, Data Type Conversion/1

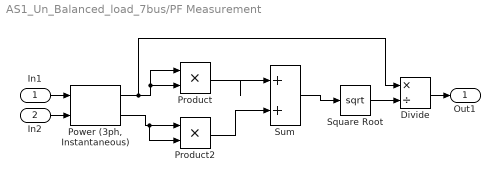
== system AS1_Un_Balanced_load_7bus/PF Measurement ==
  In1 : Inport
  In2 : Inport  Port=2
  Divide : Product  Inputs=*/
  "Power (3ph, Instantaneous)" : spsPower3phInstantaneousLib/Power (3ph, Instantaneous)
  Product : Product
  Product2 : Product
  Square Root : Sqrt  SaturateOnIntegerOverflow=on
  Sum : Sum  Inputs=|++
  Out1 : Outport  VectorParamsAs1DForOutWhenUnconnected=off
  wires:
  "Power (3ph, Instantaneous)"/1 -> Divide/1, Product/2, Product/1
  In2/1 -> "Power (3ph, Instantaneous)"/2
  Product2/1 -> Sum/2
  Sum/1 -> Square Root/1
  In1/1 -> "Power (3ph, Instantaneous)"/1
  "Power (3ph, Instantaneous)"/2 -> Product2/2, Product2/1
  Product/1 -> Sum/1
  Square Root/1 -> Divide/2
  Divide/1 -> Out1/1

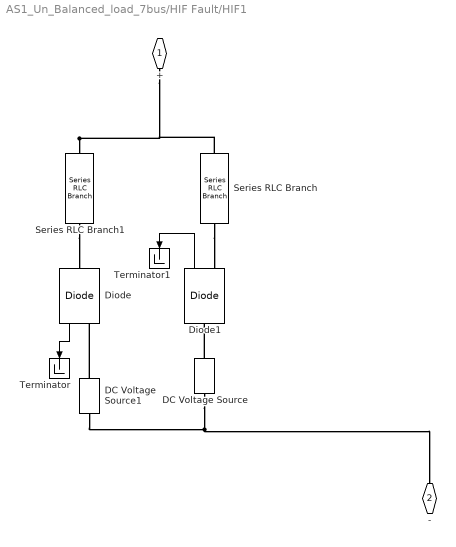
== system AS1_Un_Balanced_load_7bus/HIF Fault/HIF1 ==
  DC Voltage Source : spsDCVoltageSourceLib/DC Voltage Source  Amplitude=1800  Measurements=None
  DC Voltage Source1 : spsDCVoltageSourceLib/DC Voltage Source  Amplitude=2700  Measurements=None
  Diode : spsDiodeLib/Diode  Ron=0.001  Lon=0  Vf=0.8  IC=0  UseSnubber=off  Rs=500  Cs=250e-9  Measurements=on
  Diode1 : spsDiodeLib/Diode  Ron=0.001  Lon=0  Vf=0.8  IC=0  UseSnubber=off  Rs=500  Cs=250e-9  Measurements=on
  Series RLC Branch : spsSeriesRLCBranchLib/Series RLC Branch  LConnTagsString=__new0  RConnTagsString=__new0  BranchType=R  Resistance=500  Inductance=1e-3  SetiL0=off  InitialCurrent=0  Capacitance=1e-6  Setx0=off  InitialVoltage=0  Measurements=None
  Series RLC Branch1 : spsSeriesRLCBranchLib/Series RLC Branch  LConnTagsString=__new0  RConnTagsString=__new0  BranchType=R  Resistance=500  Inductance=1e-3  SetiL0=off  InitialCurrent=0  Capacitance=1e-6  Setx0=off  InitialVoltage=0  Measurements=None
  Terminator : Terminator
  Terminator1 : Terminator
  + : PMIOPort  Side=Left
  - : PMIOPort  Port=2  Side=Right
  wires:
  Diode/1 -> Terminator/1
  Diode1/1 -> Terminator1/1
  connections:
  Series RLC Branch1/RConn1 -- Diode/LConn1
  DC Voltage Source1/RConn1 -- Diode/RConn1
  DC Voltage Source/RConn1 -- -/RConn1 -- DC Voltage Source1/LConn1
  Series RLC Branch/RConn1 -- Diode1/RConn1
  Series RLC Branch1/LConn1 -- +/RConn1 -- Series RLC Branch/LConn1
  DC Voltage Source/LConn1 -- Diode1/LConn1

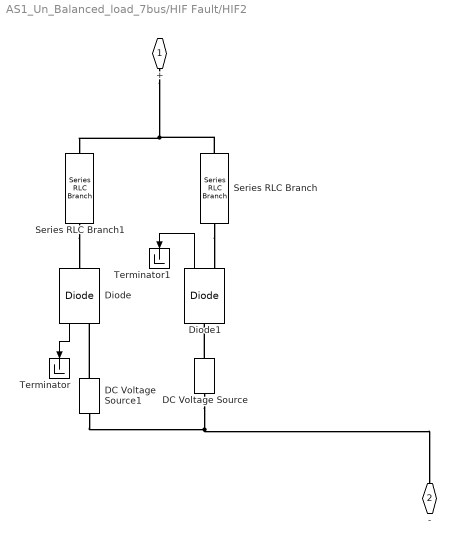
== system AS1_Un_Balanced_load_7bus/HIF Fault/HIF2 ==
  DC Voltage Source : spsDCVoltageSourceLib/DC Voltage Source  Amplitude=1800  Measurements=None
  DC Voltage Source1 : spsDCVoltageSourceLib/DC Voltage Source  Amplitude=2800  Measurements=None
  Diode : spsDiodeLib/Diode  Ron=0.001  Lon=0  Vf=0.8  IC=0  UseSnubber=off  Rs=500  Cs=250e-9  Measurements=on
  Diode1 : spsDiodeLib/Diode  Ron=0.001  Lon=0  Vf=0.8  IC=0  UseSnubber=off  Rs=500  Cs=250e-9  Measurements=on
  Series RLC Branch : spsSeriesRLCBranchLib/Series RLC Branch  LConnTagsString=__new0  RConnTagsString=__new0  BranchType=R  Resistance=520  Inductance=1e-3  SetiL0=off  InitialCurrent=0  Capacitance=1e-6  Setx0=off  InitialVoltage=0  Measurements=None
  Series RLC Branch1 : spsSeriesRLCBranchLib/Series RLC Branch  LConnTagsString=__new0  RConnTagsString=__new0  BranchType=R  Resistance=520  Inductance=1e-3  SetiL0=off  InitialCurrent=0  Capacitance=1e-6  Setx0=off  InitialVoltage=0  Measurements=None
  Terminator : Terminator
  Terminator1 : Terminator
  + : PMIOPort  Side=Left
  - : PMIOPort  Port=2  Side=Right
  wires:
  Diode/1 -> Terminator/1
  Diode1/1 -> Terminator1/1
  connections:
  Series RLC Branch1/RConn1 -- Diode/LConn1
  DC Voltage Source1/RConn1 -- Diode/RConn1
  DC Voltage Source1/LConn1 -- DC Voltage Source/RConn1 -- -/RConn1
  Series RLC Branch/RConn1 -- Diode1/RConn1
  Series RLC Branch/LConn1 -- Series RLC Branch1/LConn1 -- +/RConn1
  DC Voltage Source/LConn1 -- Diode1/LConn1

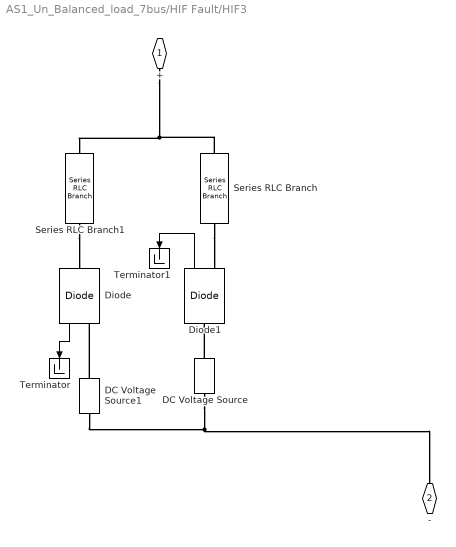
== system AS1_Un_Balanced_load_7bus/HIF Fault/HIF3 ==
  DC Voltage Source : spsDCVoltageSourceLib/DC Voltage Source  Amplitude=1900  Measurements=None
  DC Voltage Source1 : spsDCVoltageSourceLib/DC Voltage Source  Amplitude=2900  Measurements=None
  Diode : spsDiodeLib/Diode  Ron=0.001  Lon=0  Vf=0.8  IC=0  UseSnubber=off  Rs=500  Cs=250e-9  Measurements=on
  Diode1 : spsDiodeLib/Diode  Ron=0.001  Lon=0  Vf=0.8  IC=0  UseSnubber=off  Rs=500  Cs=250e-9  Measurements=on
  Series RLC Branch : spsSeriesRLCBranchLib/Series RLC Branch  LConnTagsString=__new0  RConnTagsString=__new0  BranchType=R  Resistance=540  Inductance=1e-3  SetiL0=off  InitialCurrent=0  Capacitance=1e-6  Setx0=off  InitialVoltage=0  Measurements=None
  Series RLC Branch1 : spsSeriesRLCBranchLib/Series RLC Branch  LConnTagsString=__new0  RConnTagsString=__new0  BranchType=R  Resistance=540  Inductance=1e-3  SetiL0=off  InitialCurrent=0  Capacitance=1e-6  Setx0=off  InitialVoltage=0  Measurements=None
  Terminator : Terminator
  Terminator1 : Terminator
  + : PMIOPort  Side=Left
  - : PMIOPort  Port=2  Side=Right
  wires:
  Diode/1 -> Terminator/1
  Diode1/1 -> Terminator1/1
  connections:
  Series RLC Branch1/RConn1 -- Diode/LConn1
  DC Voltage Source1/RConn1 -- Diode/RConn1
  DC Voltage Source1/LConn1 -- DC Voltage Source/RConn1 -- -/RConn1
  Series RLC Branch/RConn1 -- Diode1/RConn1
  Series RLC Branch/LConn1 -- Series RLC Branch1/LConn1 -- +/RConn1
  DC Voltage Source/LConn1 -- Diode1/LConn1

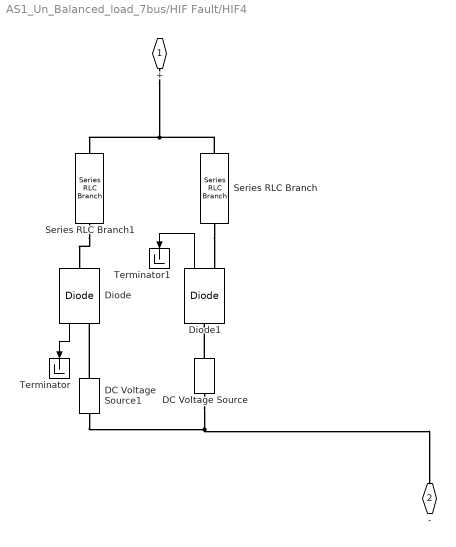
== system AS1_Un_Balanced_load_7bus/HIF Fault/HIF4 ==
  DC Voltage Source : spsDCVoltageSourceLib/DC Voltage Source  Amplitude=2000  Measurements=None
  DC Voltage Source1 : spsDCVoltageSourceLib/DC Voltage Source  Amplitude=3000  Measurements=None
  Diode : spsDiodeLib/Diode  Ron=0.001  Lon=0  Vf=0.8  IC=0  UseSnubber=off  Rs=500  Cs=250e-9  Measurements=on
  Diode1 : spsDiodeLib/Diode  Ron=0.001  Lon=0  Vf=0.8  IC=0  UseSnubber=off  Rs=500  Cs=250e-9  Measurements=on
  Series RLC Branch : spsSeriesRLCBranchLib/Series RLC Branch  LConnTagsString=__new0  RConnTagsString=__new0  BranchType=R  Resistance=560  Inductance=1e-3  SetiL0=off  InitialCurrent=0  Capacitance=1e-6  Setx0=off  InitialVoltage=0  Measurements=None
  Series RLC Branch1 : spsSeriesRLCBranchLib/Series RLC Branch  LConnTagsString=__new0  RConnTagsString=__new0  BranchType=R  Resistance=560  Inductance=1e-3  SetiL0=off  InitialCurrent=0  Capacitance=1e-6  Setx0=off  InitialVoltage=0  Measurements=None
  Terminator : Terminator
  Terminator1 : Terminator
  + : PMIOPort  Side=Left
  - : PMIOPort  Port=2  Side=Right
  wires:
  Diode/1 -> Terminator/1
  Diode1/1 -> Terminator1/1
  connections:
  Series RLC Branch1/RConn1 -- Diode/LConn1
  DC Voltage Source1/RConn1 -- Diode/RConn1
  DC Voltage Source1/LConn1 -- DC Voltage Source/RConn1 -- -/RConn1
  Series RLC Branch/RConn1 -- Diode1/RConn1
  Series RLC Branch/LConn1 -- Series RLC Branch1/LConn1 -- +/RConn1
  DC Voltage Source/LConn1 -- Diode1/LConn1

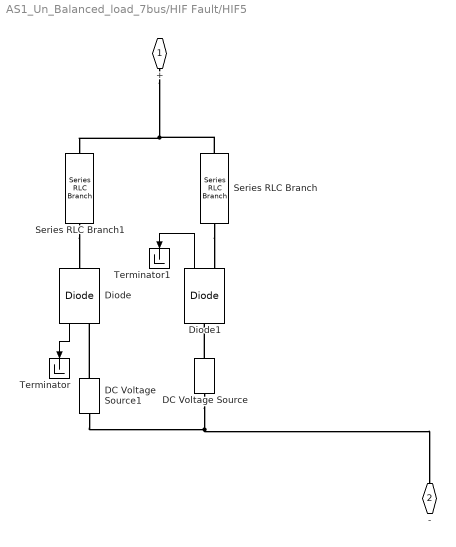
== system AS1_Un_Balanced_load_7bus/HIF Fault/HIF5 ==
  DC Voltage Source : spsDCVoltageSourceLib/DC Voltage Source  Amplitude=2100  Measurements=None
  DC Voltage Source1 : spsDCVoltageSourceLib/DC Voltage Source  Amplitude=3100  Measurements=None
  Diode : spsDiodeLib/Diode  Ron=0.001  Lon=0  Vf=0.8  IC=0  UseSnubber=off  Rs=500  Cs=250e-9  Measurements=on
  Diode1 : spsDiodeLib/Diode  Ron=0.001  Lon=0  Vf=0.8  IC=0  UseSnubber=off  Rs=500  Cs=250e-9  Measurements=on
  Series RLC Branch : spsSeriesRLCBranchLib/Series RLC Branch  LConnTagsString=__new0  RConnTagsString=__new0  BranchType=R  Resistance=580  Inductance=1e-3  SetiL0=off  InitialCurrent=0  Capacitance=1e-6  Setx0=off  InitialVoltage=0  Measurements=None
  Series RLC Branch1 : spsSeriesRLCBranchLib/Series RLC Branch  LConnTagsString=__new0  RConnTagsString=__new0  BranchType=R  Resistance=580  Inductance=1e-3  SetiL0=off  InitialCurrent=0  Capacitance=1e-6  Setx0=off  InitialVoltage=0  Measurements=None
  Terminator : Terminator
  Terminator1 : Terminator
  + : PMIOPort  Side=Left
  - : PMIOPort  Port=2  Side=Right
  wires:
  Diode/1 -> Terminator/1
  Diode1/1 -> Terminator1/1
  connections:
  Series RLC Branch1/RConn1 -- Diode/LConn1
  DC Voltage Source1/RConn1 -- Diode/RConn1
  DC Voltage Source1/LConn1 -- DC Voltage Source/RConn1 -- -/RConn1
  Series RLC Branch/RConn1 -- Diode1/RConn1
  Series RLC Branch/LConn1 -- Series RLC Branch1/LConn1 -- +/RConn1
  DC Voltage Source/LConn1 -- Diode1/LConn1

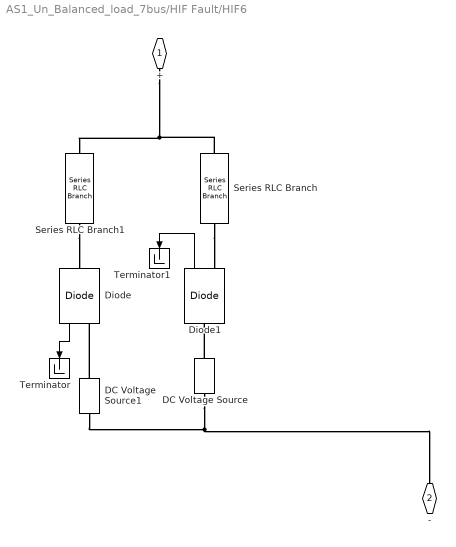
== system AS1_Un_Balanced_load_7bus/HIF Fault/HIF6 ==
  DC Voltage Source : spsDCVoltageSourceLib/DC Voltage Source  Amplitude=2200  Measurements=None
  DC Voltage Source1 : spsDCVoltageSourceLib/DC Voltage Source  Amplitude=3200  Measurements=None
  Diode : spsDiodeLib/Diode  Ron=0.001  Lon=0  Vf=0.8  IC=0  UseSnubber=off  Rs=500  Cs=250e-9  Measurements=on
  Diode1 : spsDiodeLib/Diode  Ron=0.001  Lon=0  Vf=0.8  IC=0  UseSnubber=off  Rs=500  Cs=250e-9  Measurements=on
  Series RLC Branch : spsSeriesRLCBranchLib/Series RLC Branch  LConnTagsString=__new0  RConnTagsString=__new0  BranchType=R  Resistance=600  Inductance=1e-3  SetiL0=off  InitialCurrent=0  Capacitance=1e-6  Setx0=off  InitialVoltage=0  Measurements=None
  Series RLC Branch1 : spsSeriesRLCBranchLib/Series RLC Branch  LConnTagsString=__new0  RConnTagsString=__new0  BranchType=R  Resistance=600  Inductance=1e-3  SetiL0=off  InitialCurrent=0  Capacitance=1e-6  Setx0=off  InitialVoltage=0  Measurements=None
  Terminator : Terminator
  Terminator1 : Terminator
  + : PMIOPort  Side=Left
  - : PMIOPort  Port=2  Side=Right
  wires:
  Diode/1 -> Terminator/1
  Diode1/1 -> Terminator1/1
  connections:
  Series RLC Branch1/RConn1 -- Diode/LConn1
  DC Voltage Source1/RConn1 -- Diode/RConn1
  DC Voltage Source1/LConn1 -- DC Voltage Source/RConn1 -- -/RConn1
  Series RLC Branch/RConn1 -- Diode1/RConn1
  Series RLC Branch/LConn1 -- Series RLC Branch1/LConn1 -- +/RConn1
  DC Voltage Source/LConn1 -- Diode1/LConn1

== matlab function AS1_Un_Balanced_load_7bus/MATLAB Function1 ==
  data: P input; Energy output; t input
function Energy= fcn(P,t)
Energy=P*t;
%#codegen
